simulink library "INT_RngMod_TrqFrcCalc"  (R2016b)
settings: Solver=VariableStepAuto  StartTime=0.0  StopTime=10.0  RelTol=1e-3
settings Model: Creator=Administrator  LastModifiedBy=Administrator

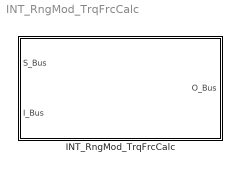
== system INT_RngMod_TrqFrcCalc ==
  INT_RngMod_TrqFrcCalc : Subsystem

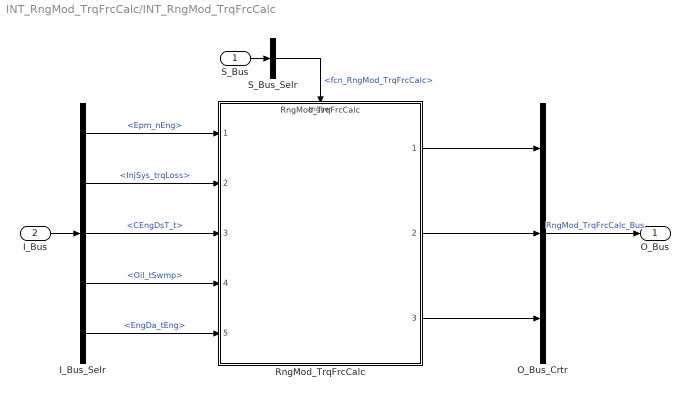
== system INT_RngMod_TrqFrcCalc/INT_RngMod_TrqFrcCalc ==
  S_Bus : Inport
  I_Bus : Inport  Port=2
  I_Bus_Selr : BusSelector  OutputSignals=Epm_nEng,InjSys_trqLoss,CEngDsT_t,Oil_tSwmp,EngDa_tEng
  O_Bus_Crtr : BusCreator  Inputs=3
  RngMod_TrqFrcCalc : ModelReference  ModelNameDialog=RngMod_TrqFrcCalc  SimulationMode=Normal  ModelReferenceVersion=1.3  TriggerPortName=function  TriggerPortTriggerType=function-call  TriggerPortStatesWhenEnabling=held
  S_Bus_Selr : BusSelector  OutputSignals=fcn_RngMod_TrqFrcCalc
  O_Bus : Outport
  wires:
  S_Bus_Selr/1 -> RngMod_TrqFrcCalc/Trigger  "<fcn_RngMod_TrqFrcCalc>"
  S_Bus/1 -> S_Bus_Selr/1
  I_Bus/1 -> I_Bus_Selr/1
  I_Bus_Selr/1 -> RngMod_TrqFrcCalc/1  "<Epm_nEng>"
  I_Bus_Selr/2 -> RngMod_TrqFrcCalc/2  "<InjSys_trqLoss>"
  I_Bus_Selr/3 -> RngMod_TrqFrcCalc/3  "<CEngDsT_t>"
  I_Bus_Selr/4 -> RngMod_TrqFrcCalc/4  "<Oil_tSwmp>"
  I_Bus_Selr/5 -> RngMod_TrqFrcCalc/5  "<EngDa_tEng>"
  O_Bus_Crtr/1 -> O_Bus/1  "RngMod_TrqFrcCalc_Bus"
  RngMod_TrqFrcCalc/1 -> O_Bus_Crtr/1
  RngMod_TrqFrcCalc/2 -> O_Bus_Crtr/2
  RngMod_TrqFrcCalc/3 -> O_Bus_Crtr/3
